simulink model "VoiceTransmission"  (R2018a)
settings: Solver=VariableStepAuto  StartTime=0.0  StopTime=10.0  RelTol=1e-3
libraries: commanabbnd3 x2, commchan3 x1, dspvision x1
settings Model: Creator=ASUS  LastModifiedBy=ASUS

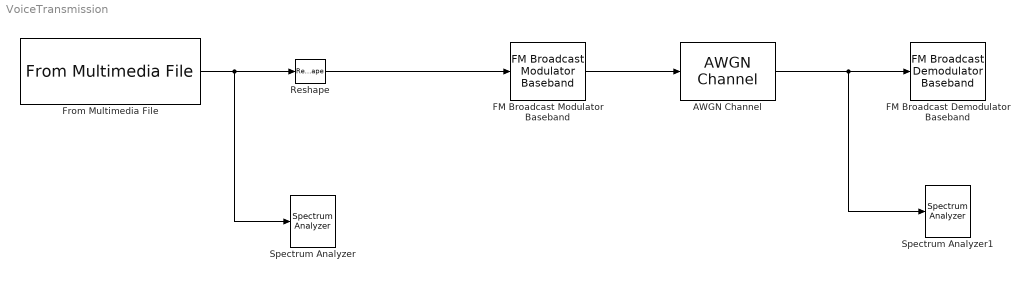
== system VoiceTransmission ==
  AWGN Channel : commchan3/AWGN Channel  InputProcessing=Columns as channels (frame based)  seed=67  noiseMode="Signal to noise ratio  (Eb/No)"  EbNodB=10  EsNodB=10  SNRdB=10  bitsPerSym=1  Ps=1  Tsym=1  variance=1
  FM Broadcast Demodulator Baseband : commanabbnd3/FM Broadcast Demodulator Baseband  SampleRate=240e3  FrequencyDeviation=75e3  FilterTimeConstant=75e-6  AudioSampleRate=48000  PlaySound=on  BufferSize=4096  Stereo=off  RBDS=off  RBDSSamplesPerSymbol=10  RBDSCostasLoop=off  SimulateUsing=Code generation
      settings: SourceProductName=Communications System Toolbox  SourceProductBaseCode=CM
  FM Broadcast Modulator Baseband : commanabbnd3/FM Broadcast Modulator Baseband  SampleRate=240e3  FrequencyDeviation=75e3  FilterTimeConstant=75e-6  AudioSampleRate=48e3  Stereo=off  RBDS=off  RBDSSamplesPerSymbol=10  SimulateUsing=Code generation
      settings: SourceProductName=Communications System Toolbox  SourceProductBaseCode=CM
  From Multimedia File : dspvision/From Multimedia File  inputFilename=C:\Program Files\MATLAB\R2018a\toolbox\dsp\dsp\dspafxf_8000.wav  loop=on  numPlays=inf  outputStreams=Audio only  videoDataType=single  audioDataType=double  inheritSampleTime=on  userDefinedSampleTime=1/30  noAudioOutput=off  isIntensityVideo=off  fourcc=RGB  colorVideoFormat=Separate color signals  outputEOF=off  dataOrg=Column-major  audioFrameSize=1024  computeAudioFrameSize=off  outSamplingMode=Sample based
      settings: SourceProductBaseCode=VP
  Reshape : Reshape
  Spectrum Analyzer : SpectrumAnalyzer
  Spectrum Analyzer1 : SpectrumAnalyzer
  wires:
  From Multimedia File/1 -> Reshape/1, Spectrum Analyzer/1
  Reshape/1 -> FM Broadcast Modulator Baseband/1
  FM Broadcast Modulator Baseband/1 -> AWGN Channel/1
  AWGN Channel/1 -> Spectrum Analyzer1/1, FM Broadcast Demodulator Baseband/1
